simulink model "check_fence"  (Simulink 7.4)
settings: Solver=ode45  StartTime=0.0  StopTime=10.0  RelTol=1e-3
libraries: xbsIndex_r4 x293
(part 1 of 2)
settings Model: Creator=andryc  LastModifiedBy=andryc

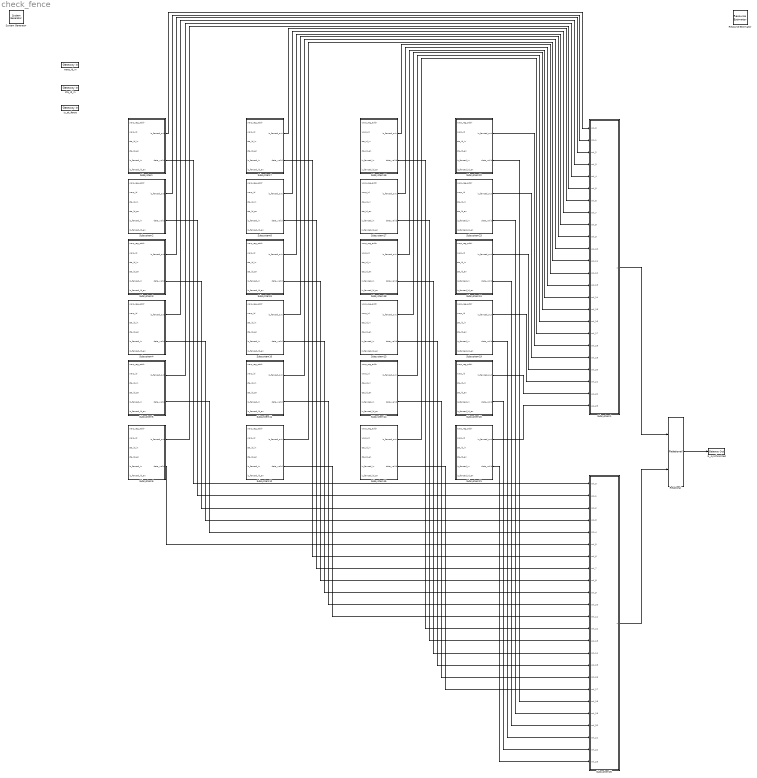
== system check_fence ==
  " System Generator" : xbsIndex_r4/ System Generator  Tag=genX  SystemSampleTime=-1  xilinxfamily=Virtex6  part=xc6vsx315t  speed=-3  package=ff1156  synthesis_tool=XST  clock_wrapper=Clock Enables  directory=./netlist  testbench=off  simulink_period=1  sysclk_period=10  dcm_input_clock_period=10  incr_netlist=off  trim_vbits=Everywhere in SubSystem  dbl_ovrd=According to Block Masks  core_generation=According to Block Masks  run_coregen=off  deprecated_control=off  eval_field=0  block_type=sysgen
  Relational : xbsIndex_r4/Relational  mode=a=b  en=off  latency=0  dbl_ovrd=off  block_type=relational
  Resource Estimator : xbsIndex_r4/Resource Estimator  Tag=resEstTag  Slices=0  FFs=0  BRAMs=0  LUTs=0  IOBs=0  EBMs=0  TBUFs=0  xl_use_estimator_area=off  est_options=Estimate  block_type=resource_estimator
      settings: AttributesFormatString=Resource\nEstimator
  Subsystem : Subsystem
  Subsystem1 : Subsystem
  Subsystem10 : Subsystem
  Subsystem11 : Subsystem
  Subsystem12 : Subsystem
  Subsystem13 : Subsystem
  Subsystem14 : Subsystem
  Subsystem15 : Subsystem
  Subsystem16 : Subsystem
  Subsystem17 : Subsystem
  Subsystem18 : Subsystem
  Subsystem19 : Subsystem
  Subsystem2 : Subsystem
  Subsystem20 : Subsystem
  Subsystem21 : Subsystem
  Subsystem22 : Subsystem
  Subsystem23 : Subsystem
  Subsystem24 : Subsystem
  Subsystem25 : Subsystem
  Subsystem3 : Subsystem
  Subsystem4 : Subsystem
  Subsystem5 : Subsystem
  Subsystem6 : Subsystem
  Subsystem7 : Subsystem
  Subsystem8 : Subsystem
  Subsystem9 : Subsystem
  cta_id_in : xbsIndex_r4/Gateway In  arith_type=Unsigned  n_bits=2  bin_pt=0  quantization=Truncate  overflow=Saturate  period=1  dbl_ovrd=off  timing_constraint=None  locs_specified=off  LOCs={}  hdl_port=on  block_type=gatewayin
      settings: infoedit="Gateway in block.  Converts inputs of type Simulink integer, double and fixed point to  Xilinx fixed point type.<br><br>Hardware notes:  In hardware these blocks become top level input ports."
  is_at_fence : xbsIndex_r4/Gateway In  arith_type=Unsigned  n_bits=2  bin_pt=0  quantization=Truncate  overflow=Saturate  period=1  dbl_ovrd=off  timing_constraint=None  locs_specified=off  LOCs={}  hdl_port=on  block_type=gatewayin
      settings: infoedit="Gateway in block.  Converts inputs of type Simulink integer, double and fixed point to  Xilinx fixed point type.<br><br>Hardware notes:  In hardware these blocks become top level input ports."
  is_synchronized : xbsIndex_r4/Gateway Out  hdl_port=on  timing_constraint=None  locs_specified=off  LOCs={}  block_type=gatewayout
      settings: infoedit="Gateway out block.  Converts Xilinx fixed point inputs into ouputs of type Simulink integer, double, or fixed point.<br><br>Hardware notes:  In hardware these blocks become top level output ports or are discarded, depending on how they are configured."
  warp_id_in : xbsIndex_r4/Gateway In  arith_type=Unsigned  n_bits=4  bin_pt=0  quantization=Truncate  overflow=Saturate  period=1  dbl_ovrd=off  timing_constraint=None  locs_specified=off  LOCs={}  hdl_port=on  block_type=gatewayin
      settings: infoedit="Gateway in block.  Converts inputs of type Simulink integer, double and fixed point to  Xilinx fixed point type.<br><br>Hardware notes:  In hardware these blocks become top level input ports."
  wires:
  Subsystem/1(is_fenced_out) -> Subsystem1/1(val_0)
  Subsystem2/1(is_fenced_out) -> Subsystem1/2(val_1)
  Subsystem3/1(is_fenced_out) -> Subsystem1/3(val_2)
  Subsystem4/1(is_fenced_out) -> Subsystem1/4(val_3)
  Subsystem5/1(is_fenced_out) -> Subsystem1/5(val_4)
  Subsystem6/1(is_fenced_out) -> Subsystem1/6(val_5)
  Subsystem7/1(is_fenced_out) -> Subsystem1/7(val_6)
  Subsystem8/1(is_fenced_out) -> Subsystem1/8(val_7)
  Subsystem9/1(is_fenced_out) -> Subsystem1/9(val_8)
  Subsystem10/1(is_fenced_out) -> Subsystem1/10(val_9)
  Subsystem11/1(is_fenced_out) -> Subsystem1/11(val_10)
  Subsystem12/1(is_fenced_out) -> Subsystem1/12(val_11)
  Subsystem16/1(is_fenced_out) -> Subsystem1/13(val_12)
  Subsystem17/1(is_fenced_out) -> Subsystem1/14(val_13)
  Subsystem18/1(is_fenced_out) -> Subsystem1/15(val_14)
  Subsystem13/1(is_fenced_out) -> Subsystem1/16(val_15)
  Subsystem14/1(is_fenced_out) -> Subsystem1/17(val_16)
  Subsystem15/1(is_fenced_out) -> Subsystem1/18(val_17)
  Subsystem22/1(is_fenced_out) -> Subsystem1/19(val_18)
  Subsystem23/1(is_fenced_out) -> Subsystem1/20(val_19)
  Subsystem24/1(is_fenced_out) -> Subsystem1/21(val_20)
  Subsystem19/1(is_fenced_out) -> Subsystem1/22(val_21)
  Subsystem20/1(is_fenced_out) -> Subsystem1/23(val_22)
  Subsystem21/1(is_fenced_out) -> Subsystem1/24(val_23)
  Subsystem/2(data_valid) -> Subsystem25/1(val_0)
  Subsystem2/2(data_valid) -> Subsystem25/2(val_1)
  Subsystem3/2(data_valid) -> Subsystem25/3(val_2)
  Subsystem4/2(data_valid) -> Subsystem25/4(val_3)
  Subsystem5/2(data_valid) -> Subsystem25/5(val_4)
  Subsystem6/2(data_valid) -> Subsystem25/6(val_5)
  Subsystem7/2(data_valid) -> Subsystem25/7(val_6)
  Subsystem8/2(data_valid) -> Subsystem25/8(val_7)
  Subsystem9/2(data_valid) -> Subsystem25/9(val_8)
  Subsystem10/2(data_valid) -> Subsystem25/10(val_9)
  Subsystem11/2(data_valid) -> Subsystem25/11(val_10)
  Subsystem12/2(data_valid) -> Subsystem25/12(val_11)
  Subsystem16/2(data_valid) -> Subsystem25/13(val_12)
  Subsystem17/2(data_valid) -> Subsystem25/14(val_13)
  Subsystem18/2(data_valid) -> Subsystem25/15(val_14)
  Subsystem13/2(data_valid) -> Subsystem25/16(val_15)
  Subsystem14/2(data_valid) -> Subsystem25/17(val_16)
  Subsystem15/2(data_valid) -> Subsystem25/18(val_17)
  Subsystem22/2(data_valid) -> Subsystem25/19(val_18)
  Subsystem23/2(data_valid) -> Subsystem25/20(val_19)
  Subsystem24/2(data_valid) -> Subsystem25/21(val_20)
  Subsystem19/2(data_valid) -> Subsystem25/22(val_21)
  Subsystem20/2(data_valid) -> Subsystem25/23(val_22)
  Subsystem21/2(data_valid) -> Subsystem25/24(val_23)
  Subsystem1/1(s) -> Relational/1
  Subsystem25/1(s) -> Relational/2
  Relational/1 -> is_synchronized/1

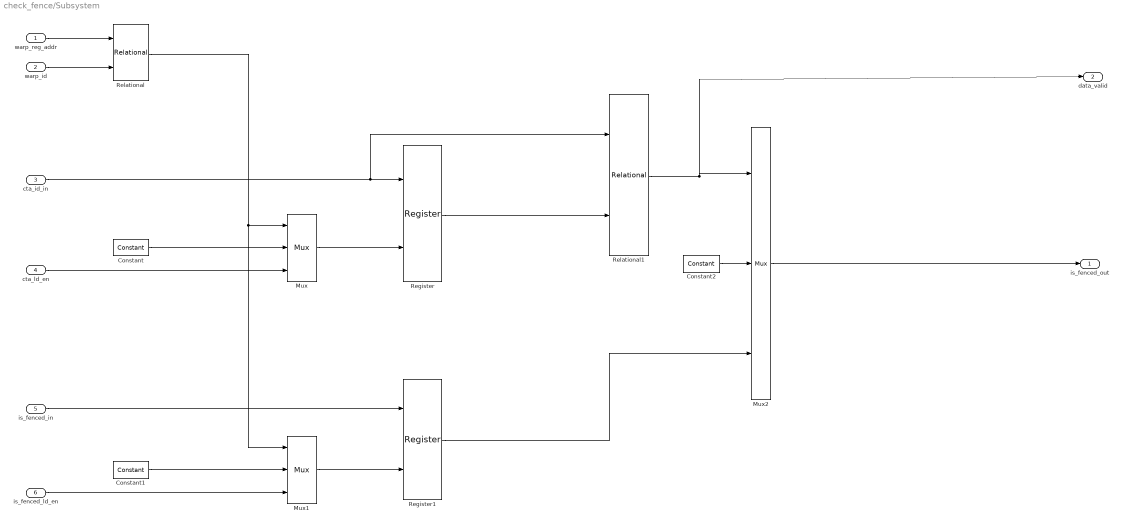
== system check_fence/Subsystem ==
  warp_reg_addr : Inport
  warp_id : Inport  Port=2
  cta_id_in : Inport  Port=3
  cta_ld_en : Inport  Port=4
  is_fenced_in : Inport  Port=5
  is_fenced_ld_en : Inport  Port=6
  Constant : xbsIndex_r4/Constant  arith_type=Boolean  const=0  n_bits=16  bin_pt=14  explicit_period=off  period=1  equ=P=C  opselect=C  inp2=PCIN>>17  opr=+  inp1=P  carry=CIN  dbl_ovrd=off  block_type=constant
  Constant1 : xbsIndex_r4/Constant  arith_type=Boolean  const=0  n_bits=16  bin_pt=14  explicit_period=off  period=1  equ=P=C  opselect=C  inp2=PCIN>>17  opr=+  inp1=P  carry=CIN  dbl_ovrd=off  block_type=constant
  Constant2 : xbsIndex_r4/Constant  arith_type=Unsigned  const=0  n_bits=1  bin_pt=0  explicit_period=off  period=1  equ=P=C  opselect=C  inp2=PCIN>>17  opr=+  inp1=P  carry=CIN  dbl_ovrd=off  block_type=constant
  Mux : xbsIndex_r4/Mux  inputs=2  en=off  latency=0  precision=Full  arith_type=Unsigned  n_bits=16  bin_pt=14  quantization=Truncate  overflow=Wrap  dbl_ovrd=off  block_type=mux
  Mux1 : xbsIndex_r4/Mux  inputs=2  en=off  latency=0  precision=Full  arith_type=Unsigned  n_bits=16  bin_pt=14  quantization=Truncate  overflow=Wrap  dbl_ovrd=off  block_type=mux
  Mux2 : xbsIndex_r4/Mux  inputs=2  en=off  latency=0  precision=Full  arith_type=Unsigned  n_bits=16  bin_pt=14  quantization=Truncate  overflow=Wrap  dbl_ovrd=off  block_type=mux
  Register : xbsIndex_r4/Register  init=0  rst=off  en=on  dbl_ovrd=off  block_type=register
  Register1 : xbsIndex_r4/Register  init=0  rst=off  en=on  dbl_ovrd=off  block_type=register
  Relational : xbsIndex_r4/Relational  mode=a=b  en=off  latency=0  dbl_ovrd=off  block_type=relational
  Relational1 : xbsIndex_r4/Relational  mode=a=b  en=off  latency=0  dbl_ovrd=off  block_type=relational
  is_fenced_out : Outport
  data_valid : Outport  Port=2
  wires:
  cta_id_in/1 -> Register/1, Relational1/1
  is_fenced_in/1 -> Register1/1
  warp_reg_addr/1 -> Relational/1
  warp_id/1 -> Relational/2
  Mux/1 -> Register/2
  cta_ld_en/1 -> Mux/3
  Constant/1 -> Mux/2
  Relational/1 -> Mux/1, Mux1/1
  Mux1/1 -> Register1/2
  is_fenced_ld_en/1 -> Mux1/3
  Constant1/1 -> Mux1/2
  Relational1/1 -> Mux2/1, data_valid/1
  Constant2/1 -> Mux2/2
  Register/1 -> Relational1/2
  Register1/1 -> Mux2/3
  Mux2/1 -> is_fenced_out/1

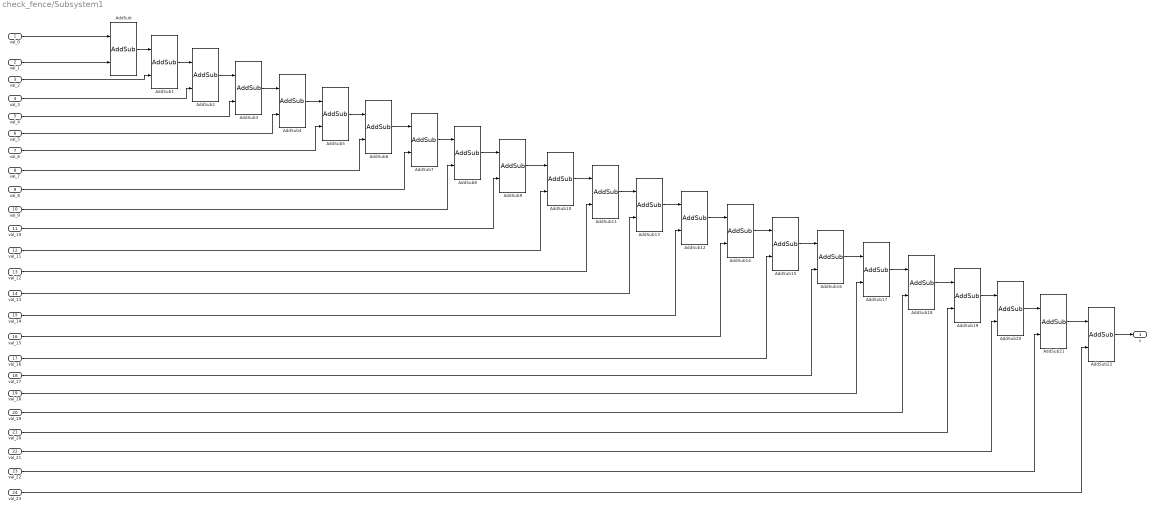
== system check_fence/Subsystem1 ==
  val_0 : Inport
  val_1 : Inport  Port=2
  val_2 : Inport  Port=3
  val_3 : Inport  Port=4
  val_4 : Inport  Port=5
  val_5 : Inport  Port=6
  val_6 : Inport  Port=7
  val_7 : Inport  Port=8
  val_8 : Inport  Port=9
  val_9 : Inport  Port=10
  val_10 : Inport  Port=11
  val_11 : Inport  Port=12
  val_12 : Inport  Port=13
  val_13 : Inport  Port=14
  val_14 : Inport  Port=15
  val_15 : Inport  Port=16
  val_16 : Inport  Port=17
  val_17 : Inport  Port=18
  val_18 : Inport  Port=19
  val_19 : Inport  Port=20
  val_20 : Inport  Port=21
  val_21 : Inport  Port=22
  val_22 : Inport  Port=23
  val_23 : Inport  Port=24
  AddSub{,1..22} (23 alike) : xbsIndex_r4/AddSub  mode=Addition  use_carryin=off  use_carryout=off  en=off  latency=0  precision=Full  arith_type=Unsigned  n_bits=16  bin_pt=14  quantization=Truncate  overflow=Wrap  dbl_ovrd=off  use_behavioral_HDL=off  hw_selection=Fabric  pipelined=off  block_type=addsub
  s : Outport
  wires:
  val_0/1 -> AddSub/1
  val_1/1 -> AddSub/2
  AddSub/1 -> AddSub1/1
  AddSub1/1 -> AddSub2/1
  AddSub2/1 -> AddSub3/1
  AddSub3/1 -> AddSub4/1
  AddSub4/1 -> AddSub5/1
  AddSub5/1 -> AddSub6/1
  AddSub6/1 -> AddSub7/1
  AddSub7/1 -> AddSub8/1
  AddSub8/1 -> AddSub9/1
  AddSub9/1 -> AddSub10/1
  AddSub10/1 -> AddSub11/1
  AddSub11/1 -> AddSub13/1
  AddSub13/1 -> AddSub12/1
  AddSub12/1 -> AddSub14/1
  AddSub14/1 -> AddSub15/1
  AddSub15/1 -> AddSub16/1
  AddSub16/1 -> AddSub17/1
  AddSub17/1 -> AddSub18/1
  AddSub18/1 -> AddSub19/1
  AddSub19/1 -> AddSub20/1
  AddSub20/1 -> AddSub21/1
  AddSub21/1 -> AddSub22/1
  AddSub22/1 -> s/1
  val_2/1 -> AddSub1/2
  val_3/1 -> AddSub2/2
  val_4/1 -> AddSub3/2
  val_5/1 -> AddSub4/2
  val_6/1 -> AddSub5/2
  val_7/1 -> AddSub6/2
  val_8/1 -> AddSub7/2
  val_9/1 -> AddSub8/2
  val_10/1 -> AddSub9/2
  val_11/1 -> AddSub10/2
  val_12/1 -> AddSub11/2
  val_13/1 -> AddSub13/2
  val_14/1 -> AddSub12/2
  val_15/1 -> AddSub14/2
  val_16/1 -> AddSub15/2
  val_17/1 -> AddSub16/2
  val_18/1 -> AddSub17/2
  val_19/1 -> AddSub18/2
  val_20/1 -> AddSub19/2
  val_21/1 -> AddSub20/2
  val_22/1 -> AddSub21/2
  val_23/1 -> AddSub22/2

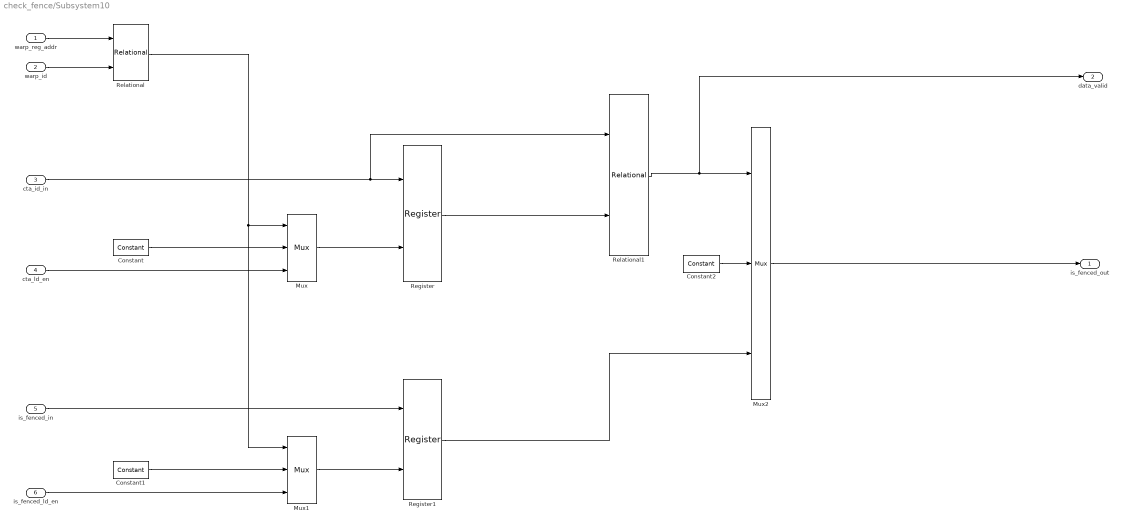
== system check_fence/Subsystem10 ==
  warp_reg_addr : Inport
  warp_id : Inport  Port=2
  cta_id_in : Inport  Port=3
  cta_ld_en : Inport  Port=4
  is_fenced_in : Inport  Port=5
  is_fenced_ld_en : Inport  Port=6
  Constant : xbsIndex_r4/Constant  arith_type=Boolean  const=0  n_bits=16  bin_pt=14  explicit_period=off  period=1  equ=P=C  opselect=C  inp2=PCIN>>17  opr=+  inp1=P  carry=CIN  dbl_ovrd=off  block_type=constant
  Constant1 : xbsIndex_r4/Constant  arith_type=Boolean  const=0  n_bits=16  bin_pt=14  explicit_period=off  period=1  equ=P=C  opselect=C  inp2=PCIN>>17  opr=+  inp1=P  carry=CIN  dbl_ovrd=off  block_type=constant
  Constant2 : xbsIndex_r4/Constant  arith_type=Unsigned  const=0  n_bits=1  bin_pt=0  explicit_period=off  period=1  equ=P=C  opselect=C  inp2=PCIN>>17  opr=+  inp1=P  carry=CIN  dbl_ovrd=off  block_type=constant
  Mux : xbsIndex_r4/Mux  inputs=2  en=off  latency=0  precision=Full  arith_type=Unsigned  n_bits=16  bin_pt=14  quantization=Truncate  overflow=Wrap  dbl_ovrd=off  block_type=mux
  Mux1 : xbsIndex_r4/Mux  inputs=2  en=off  latency=0  precision=Full  arith_type=Unsigned  n_bits=16  bin_pt=14  quantization=Truncate  overflow=Wrap  dbl_ovrd=off  block_type=mux
  Mux2 : xbsIndex_r4/Mux  inputs=2  en=off  latency=0  precision=Full  arith_type=Unsigned  n_bits=16  bin_pt=14  quantization=Truncate  overflow=Wrap  dbl_ovrd=off  block_type=mux
  Register : xbsIndex_r4/Register  init=0  rst=off  en=on  dbl_ovrd=off  block_type=register
  Register1 : xbsIndex_r4/Register  init=0  rst=off  en=on  dbl_ovrd=off  block_type=register
  Relational : xbsIndex_r4/Relational  mode=a=b  en=off  latency=0  dbl_ovrd=off  block_type=relational
  Relational1 : xbsIndex_r4/Relational  mode=a=b  en=off  latency=0  dbl_ovrd=off  block_type=relational
  is_fenced_out : Outport
  data_valid : Outport  Port=2
  wires:
  cta_id_in/1 -> Register/1, Relational1/1
  is_fenced_in/1 -> Register1/1
  warp_reg_addr/1 -> Relational/1
  warp_id/1 -> Relational/2
  Mux/1 -> Register/2
  cta_ld_en/1 -> Mux/3
  Constant/1 -> Mux/2
  Relational/1 -> Mux/1, Mux1/1
  Mux1/1 -> Register1/2
  is_fenced_ld_en/1 -> Mux1/3
  Constant1/1 -> Mux1/2
  Relational1/1 -> Mux2/1, data_valid/1
  Constant2/1 -> Mux2/2
  Register/1 -> Relational1/2
  Register1/1 -> Mux2/3
  Mux2/1 -> is_fenced_out/1

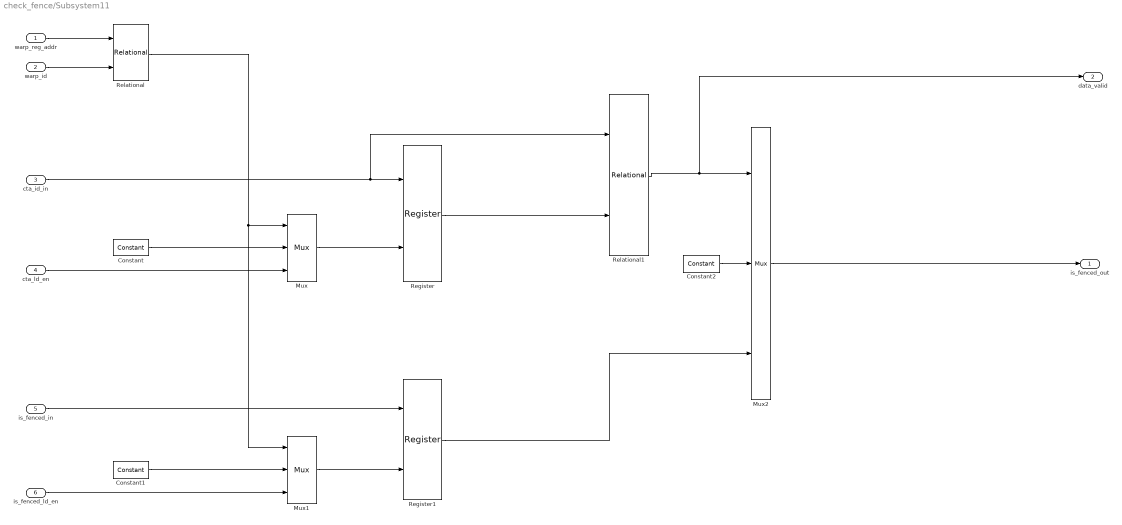
== system check_fence/Subsystem11 ==
  warp_reg_addr : Inport
  warp_id : Inport  Port=2
  cta_id_in : Inport  Port=3
  cta_ld_en : Inport  Port=4
  is_fenced_in : Inport  Port=5
  is_fenced_ld_en : Inport  Port=6
  Constant : xbsIndex_r4/Constant  arith_type=Boolean  const=0  n_bits=16  bin_pt=14  explicit_period=off  period=1  equ=P=C  opselect=C  inp2=PCIN>>17  opr=+  inp1=P  carry=CIN  dbl_ovrd=off  block_type=constant
  Constant1 : xbsIndex_r4/Constant  arith_type=Boolean  const=0  n_bits=16  bin_pt=14  explicit_period=off  period=1  equ=P=C  opselect=C  inp2=PCIN>>17  opr=+  inp1=P  carry=CIN  dbl_ovrd=off  block_type=constant
  Constant2 : xbsIndex_r4/Constant  arith_type=Unsigned  const=0  n_bits=1  bin_pt=0  explicit_period=off  period=1  equ=P=C  opselect=C  inp2=PCIN>>17  opr=+  inp1=P  carry=CIN  dbl_ovrd=off  block_type=constant
  Mux : xbsIndex_r4/Mux  inputs=2  en=off  latency=0  precision=Full  arith_type=Unsigned  n_bits=16  bin_pt=14  quantization=Truncate  overflow=Wrap  dbl_ovrd=off  block_type=mux
  Mux1 : xbsIndex_r4/Mux  inputs=2  en=off  latency=0  precision=Full  arith_type=Unsigned  n_bits=16  bin_pt=14  quantization=Truncate  overflow=Wrap  dbl_ovrd=off  block_type=mux
  Mux2 : xbsIndex_r4/Mux  inputs=2  en=off  latency=0  precision=Full  arith_type=Unsigned  n_bits=16  bin_pt=14  quantization=Truncate  overflow=Wrap  dbl_ovrd=off  block_type=mux
  Register : xbsIndex_r4/Register  init=0  rst=off  en=on  dbl_ovrd=off  block_type=register
  Register1 : xbsIndex_r4/Register  init=0  rst=off  en=on  dbl_ovrd=off  block_type=register
  Relational : xbsIndex_r4/Relational  mode=a=b  en=off  latency=0  dbl_ovrd=off  block_type=relational
  Relational1 : xbsIndex_r4/Relational  mode=a=b  en=off  latency=0  dbl_ovrd=off  block_type=relational
  is_fenced_out : Outport
  data_valid : Outport  Port=2
  wires:
  Mux2/1 -> is_fenced_out/1
  Register1/1 -> Mux2/3
  Register/1 -> Relational1/2
  Constant2/1 -> Mux2/2
  Relational1/1 -> data_valid/1, Mux2/1
  Constant1/1 -> Mux1/2
  is_fenced_ld_en/1 -> Mux1/3
  Mux1/1 -> Register1/2
  Relational/1 -> Mux1/1, Mux/1
  Constant/1 -> Mux/2
  cta_ld_en/1 -> Mux/3
  Mux/1 -> Register/2
  warp_id/1 -> Relational/2
  warp_reg_addr/1 -> Relational/1
  is_fenced_in/1 -> Register1/1
  cta_id_in/1 -> Relational1/1, Register/1

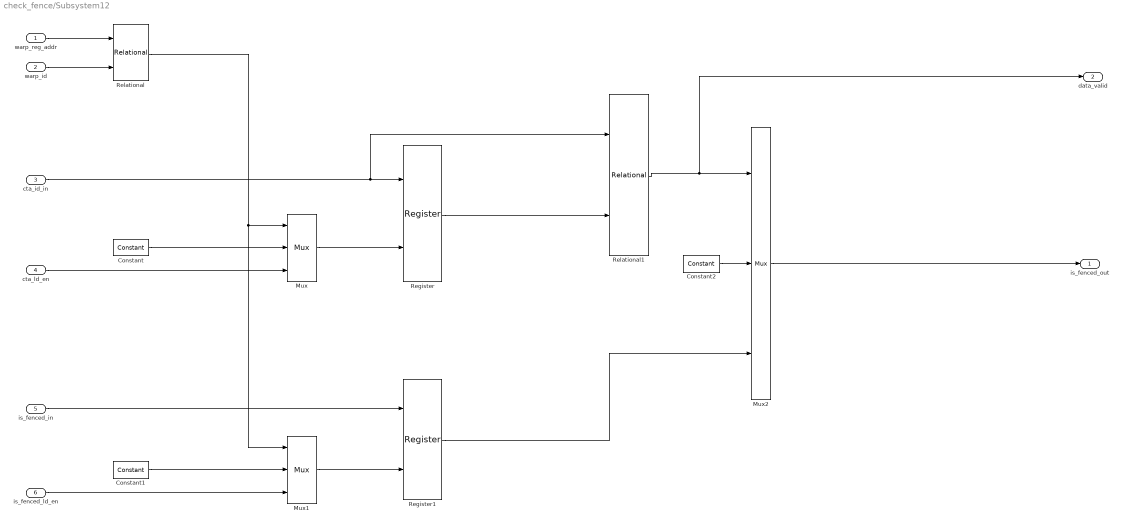
== system check_fence/Subsystem12 ==
  warp_reg_addr : Inport
  warp_id : Inport  Port=2
  cta_id_in : Inport  Port=3
  cta_ld_en : Inport  Port=4
  is_fenced_in : Inport  Port=5
  is_fenced_ld_en : Inport  Port=6
  Constant : xbsIndex_r4/Constant  arith_type=Boolean  const=0  n_bits=16  bin_pt=14  explicit_period=off  period=1  equ=P=C  opselect=C  inp2=PCIN>>17  opr=+  inp1=P  carry=CIN  dbl_ovrd=off  block_type=constant
  Constant1 : xbsIndex_r4/Constant  arith_type=Boolean  const=0  n_bits=16  bin_pt=14  explicit_period=off  period=1  equ=P=C  opselect=C  inp2=PCIN>>17  opr=+  inp1=P  carry=CIN  dbl_ovrd=off  block_type=constant
  Constant2 : xbsIndex_r4/Constant  arith_type=Unsigned  const=0  n_bits=1  bin_pt=0  explicit_period=off  period=1  equ=P=C  opselect=C  inp2=PCIN>>17  opr=+  inp1=P  carry=CIN  dbl_ovrd=off  block_type=constant
  Mux : xbsIndex_r4/Mux  inputs=2  en=off  latency=0  precision=Full  arith_type=Unsigned  n_bits=16  bin_pt=14  quantization=Truncate  overflow=Wrap  dbl_ovrd=off  block_type=mux
  Mux1 : xbsIndex_r4/Mux  inputs=2  en=off  latency=0  precision=Full  arith_type=Unsigned  n_bits=16  bin_pt=14  quantization=Truncate  overflow=Wrap  dbl_ovrd=off  block_type=mux
  Mux2 : xbsIndex_r4/Mux  inputs=2  en=off  latency=0  precision=Full  arith_type=Unsigned  n_bits=16  bin_pt=14  quantization=Truncate  overflow=Wrap  dbl_ovrd=off  block_type=mux
  Register : xbsIndex_r4/Register  init=0  rst=off  en=on  dbl_ovrd=off  block_type=register
  Register1 : xbsIndex_r4/Register  init=0  rst=off  en=on  dbl_ovrd=off  block_type=register
  Relational : xbsIndex_r4/Relational  mode=a=b  en=off  latency=0  dbl_ovrd=off  block_type=relational
  Relational1 : xbsIndex_r4/Relational  mode=a=b  en=off  latency=0  dbl_ovrd=off  block_type=relational
  is_fenced_out : Outport
  data_valid : Outport  Port=2
  wires:
  cta_id_in/1 -> Register/1, Relational1/1
  is_fenced_in/1 -> Register1/1
  warp_reg_addr/1 -> Relational/1
  warp_id/1 -> Relational/2
  Mux/1 -> Register/2
  cta_ld_en/1 -> Mux/3
  Constant/1 -> Mux/2
  Relational/1 -> Mux/1, Mux1/1
  Mux1/1 -> Register1/2
  is_fenced_ld_en/1 -> Mux1/3
  Constant1/1 -> Mux1/2
  Relational1/1 -> Mux2/1, data_valid/1
  Constant2/1 -> Mux2/2
  Register/1 -> Relational1/2
  Register1/1 -> Mux2/3
  Mux2/1 -> is_fenced_out/1

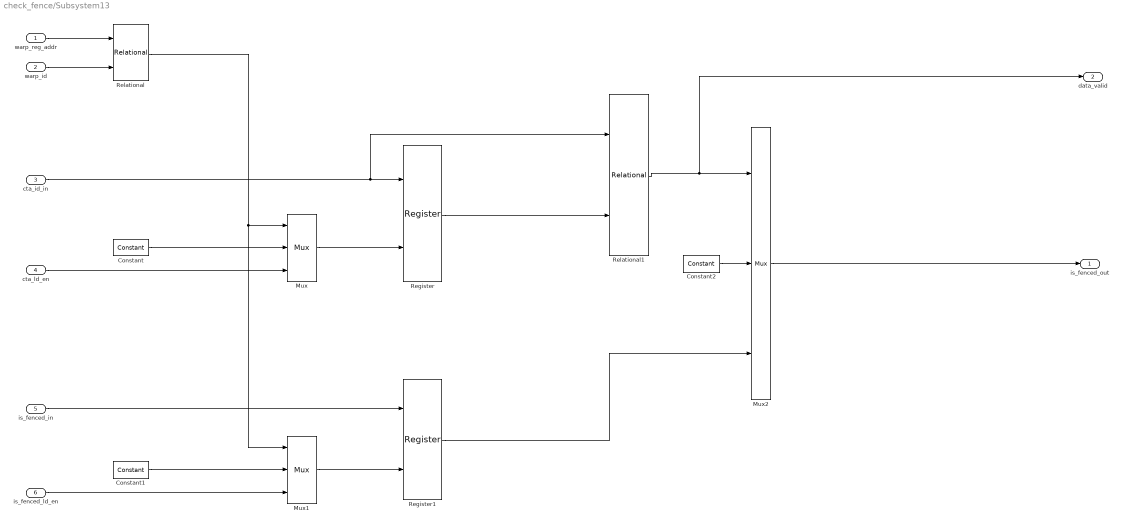
== system check_fence/Subsystem13 ==
  warp_reg_addr : Inport
  warp_id : Inport  Port=2
  cta_id_in : Inport  Port=3
  cta_ld_en : Inport  Port=4
  is_fenced_in : Inport  Port=5
  is_fenced_ld_en : Inport  Port=6
  Constant : xbsIndex_r4/Constant  arith_type=Boolean  const=0  n_bits=16  bin_pt=14  explicit_period=off  period=1  equ=P=C  opselect=C  inp2=PCIN>>17  opr=+  inp1=P  carry=CIN  dbl_ovrd=off  block_type=constant
  Constant1 : xbsIndex_r4/Constant  arith_type=Boolean  const=0  n_bits=16  bin_pt=14  explicit_period=off  period=1  equ=P=C  opselect=C  inp2=PCIN>>17  opr=+  inp1=P  carry=CIN  dbl_ovrd=off  block_type=constant
  Constant2 : xbsIndex_r4/Constant  arith_type=Unsigned  const=0  n_bits=1  bin_pt=0  explicit_period=off  period=1  equ=P=C  opselect=C  inp2=PCIN>>17  opr=+  inp1=P  carry=CIN  dbl_ovrd=off  block_type=constant
  Mux : xbsIndex_r4/Mux  inputs=2  en=off  latency=0  precision=Full  arith_type=Unsigned  n_bits=16  bin_pt=14  quantization=Truncate  overflow=Wrap  dbl_ovrd=off  block_type=mux
  Mux1 : xbsIndex_r4/Mux  inputs=2  en=off  latency=0  precision=Full  arith_type=Unsigned  n_bits=16  bin_pt=14  quantization=Truncate  overflow=Wrap  dbl_ovrd=off  block_type=mux
  Mux2 : xbsIndex_r4/Mux  inputs=2  en=off  latency=0  precision=Full  arith_type=Unsigned  n_bits=16  bin_pt=14  quantization=Truncate  overflow=Wrap  dbl_ovrd=off  block_type=mux
  Register : xbsIndex_r4/Register  init=0  rst=off  en=on  dbl_ovrd=off  block_type=register
  Register1 : xbsIndex_r4/Register  init=0  rst=off  en=on  dbl_ovrd=off  block_type=register
  Relational : xbsIndex_r4/Relational  mode=a=b  en=off  latency=0  dbl_ovrd=off  block_type=relational
  Relational1 : xbsIndex_r4/Relational  mode=a=b  en=off  latency=0  dbl_ovrd=off  block_type=relational
  is_fenced_out : Outport
  data_valid : Outport  Port=2
  wires:
  Mux2/1 -> is_fenced_out/1
  Register1/1 -> Mux2/3
  Register/1 -> Relational1/2
  Constant2/1 -> Mux2/2
  Relational1/1 -> data_valid/1, Mux2/1
  Constant1/1 -> Mux1/2
  is_fenced_ld_en/1 -> Mux1/3
  Mux1/1 -> Register1/2
  Relational/1 -> Mux1/1, Mux/1
  Constant/1 -> Mux/2
  cta_ld_en/1 -> Mux/3
  Mux/1 -> Register/2
  warp_id/1 -> Relational/2
  warp_reg_addr/1 -> Relational/1
  is_fenced_in/1 -> Register1/1
  cta_id_in/1 -> Relational1/1, Register/1

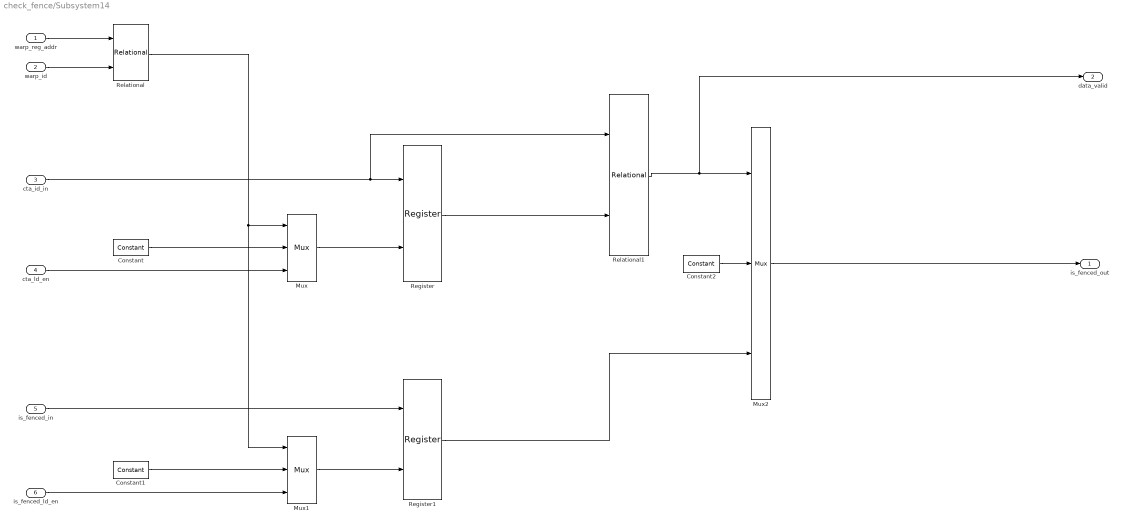
== system check_fence/Subsystem14 ==
  warp_reg_addr : Inport
  warp_id : Inport  Port=2
  cta_id_in : Inport  Port=3
  cta_ld_en : Inport  Port=4
  is_fenced_in : Inport  Port=5
  is_fenced_ld_en : Inport  Port=6
  Constant : xbsIndex_r4/Constant  arith_type=Boolean  const=0  n_bits=16  bin_pt=14  explicit_period=off  period=1  equ=P=C  opselect=C  inp2=PCIN>>17  opr=+  inp1=P  carry=CIN  dbl_ovrd=off  block_type=constant
  Constant1 : xbsIndex_r4/Constant  arith_type=Boolean  const=0  n_bits=16  bin_pt=14  explicit_period=off  period=1  equ=P=C  opselect=C  inp2=PCIN>>17  opr=+  inp1=P  carry=CIN  dbl_ovrd=off  block_type=constant
  Constant2 : xbsIndex_r4/Constant  arith_type=Unsigned  const=0  n_bits=1  bin_pt=0  explicit_period=off  period=1  equ=P=C  opselect=C  inp2=PCIN>>17  opr=+  inp1=P  carry=CIN  dbl_ovrd=off  block_type=constant
  Mux : xbsIndex_r4/Mux  inputs=2  en=off  latency=0  precision=Full  arith_type=Unsigned  n_bits=16  bin_pt=14  quantization=Truncate  overflow=Wrap  dbl_ovrd=off  block_type=mux
  Mux1 : xbsIndex_r4/Mux  inputs=2  en=off  latency=0  precision=Full  arith_type=Unsigned  n_bits=16  bin_pt=14  quantization=Truncate  overflow=Wrap  dbl_ovrd=off  block_type=mux
  Mux2 : xbsIndex_r4/Mux  inputs=2  en=off  latency=0  precision=Full  arith_type=Unsigned  n_bits=16  bin_pt=14  quantization=Truncate  overflow=Wrap  dbl_ovrd=off  block_type=mux
  Register : xbsIndex_r4/Register  init=0  rst=off  en=on  dbl_ovrd=off  block_type=register
  Register1 : xbsIndex_r4/Register  init=0  rst=off  en=on  dbl_ovrd=off  block_type=register
  Relational : xbsIndex_r4/Relational  mode=a=b  en=off  latency=0  dbl_ovrd=off  block_type=relational
  Relational1 : xbsIndex_r4/Relational  mode=a=b  en=off  latency=0  dbl_ovrd=off  block_type=relational
  is_fenced_out : Outport
  data_valid : Outport  Port=2
  wires:
  cta_id_in/1 -> Register/1, Relational1/1
  is_fenced_in/1 -> Register1/1
  warp_reg_addr/1 -> Relational/1
  warp_id/1 -> Relational/2
  Mux/1 -> Register/2
  cta_ld_en/1 -> Mux/3
  Constant/1 -> Mux/2
  Relational/1 -> Mux/1, Mux1/1
  Mux1/1 -> Register1/2
  is_fenced_ld_en/1 -> Mux1/3
  Constant1/1 -> Mux1/2
  Relational1/1 -> Mux2/1, data_valid/1
  Constant2/1 -> Mux2/2
  Register/1 -> Relational1/2
  Register1/1 -> Mux2/3
  Mux2/1 -> is_fenced_out/1

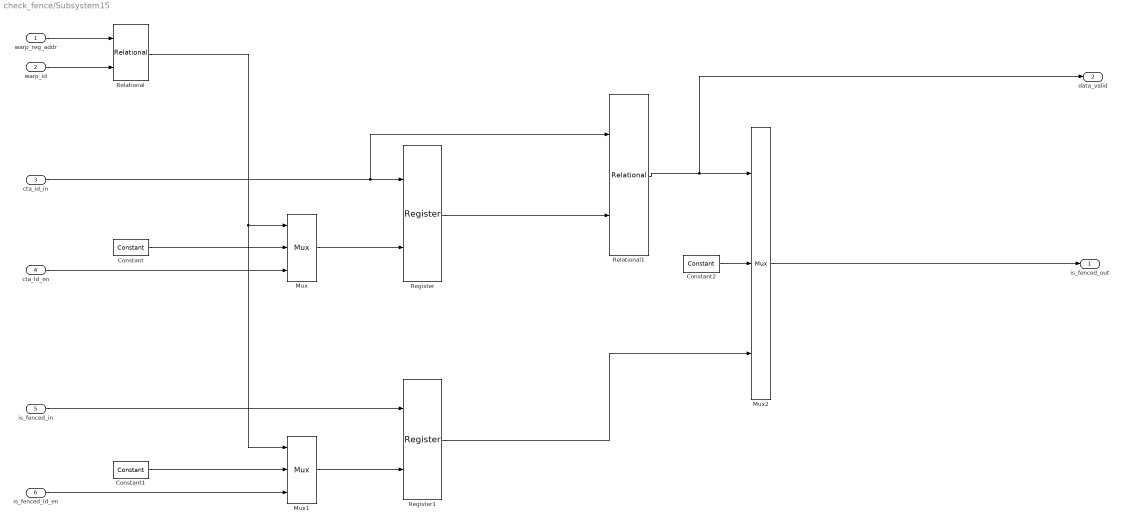
== system check_fence/Subsystem15 ==
  warp_reg_addr : Inport
  warp_id : Inport  Port=2
  cta_id_in : Inport  Port=3
  cta_ld_en : Inport  Port=4
  is_fenced_in : Inport  Port=5
  is_fenced_ld_en : Inport  Port=6
  Constant : xbsIndex_r4/Constant  arith_type=Boolean  const=0  n_bits=16  bin_pt=14  explicit_period=off  period=1  equ=P=C  opselect=C  inp2=PCIN>>17  opr=+  inp1=P  carry=CIN  dbl_ovrd=off  block_type=constant
  Constant1 : xbsIndex_r4/Constant  arith_type=Boolean  const=0  n_bits=16  bin_pt=14  explicit_period=off  period=1  equ=P=C  opselect=C  inp2=PCIN>>17  opr=+  inp1=P  carry=CIN  dbl_ovrd=off  block_type=constant
  Constant2 : xbsIndex_r4/Constant  arith_type=Unsigned  const=0  n_bits=1  bin_pt=0  explicit_period=off  period=1  equ=P=C  opselect=C  inp2=PCIN>>17  opr=+  inp1=P  carry=CIN  dbl_ovrd=off  block_type=constant
  Mux : xbsIndex_r4/Mux  inputs=2  en=off  latency=0  precision=Full  arith_type=Unsigned  n_bits=16  bin_pt=14  quantization=Truncate  overflow=Wrap  dbl_ovrd=off  block_type=mux
  Mux1 : xbsIndex_r4/Mux  inputs=2  en=off  latency=0  precision=Full  arith_type=Unsigned  n_bits=16  bin_pt=14  quantization=Truncate  overflow=Wrap  dbl_ovrd=off  block_type=mux
  Mux2 : xbsIndex_r4/Mux  inputs=2  en=off  latency=0  precision=Full  arith_type=Unsigned  n_bits=16  bin_pt=14  quantization=Truncate  overflow=Wrap  dbl_ovrd=off  block_type=mux
  Register : xbsIndex_r4/Register  init=0  rst=off  en=on  dbl_ovrd=off  block_type=register
  Register1 : xbsIndex_r4/Register  init=0  rst=off  en=on  dbl_ovrd=off  block_type=register
  Relational : xbsIndex_r4/Relational  mode=a=b  en=off  latency=0  dbl_ovrd=off  block_type=relational
  Relational1 : xbsIndex_r4/Relational  mode=a=b  en=off  latency=0  dbl_ovrd=off  block_type=relational
  is_fenced_out : Outport
  data_valid : Outport  Port=2
  wires:
  Mux2/1 -> is_fenced_out/1
  Register1/1 -> Mux2/3
  Register/1 -> Relational1/2
  Constant2/1 -> Mux2/2
  Relational1/1 -> data_valid/1, Mux2/1
  Constant1/1 -> Mux1/2
  is_fenced_ld_en/1 -> Mux1/3
  Mux1/1 -> Register1/2
  Relational/1 -> Mux1/1, Mux/1
  Constant/1 -> Mux/2
  cta_ld_en/1 -> Mux/3
  Mux/1 -> Register/2
  warp_id/1 -> Relational/2
  warp_reg_addr/1 -> Relational/1
  is_fenced_in/1 -> Register1/1
  cta_id_in/1 -> Relational1/1, Register/1

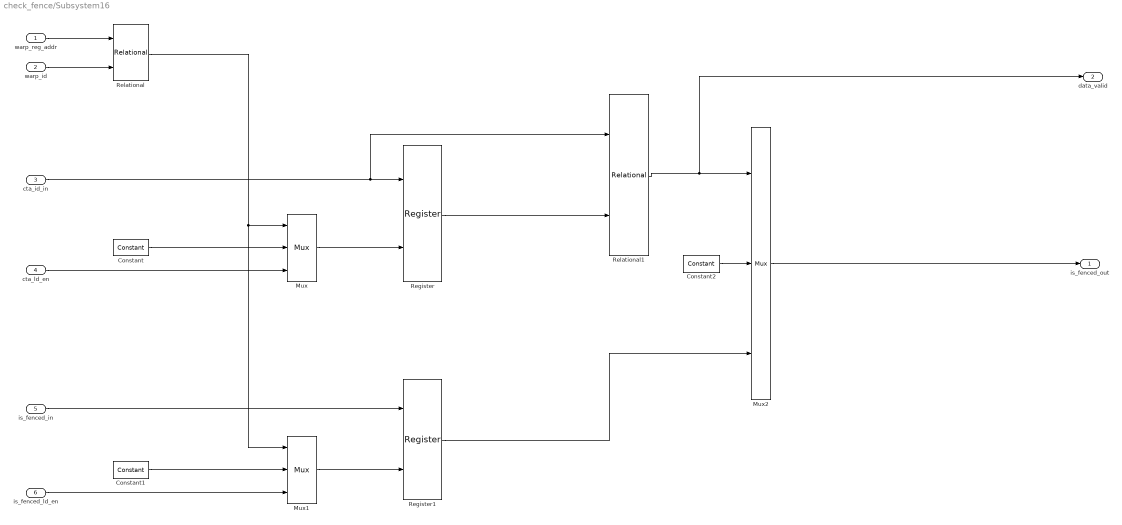
== system check_fence/Subsystem16 ==
  warp_reg_addr : Inport
  warp_id : Inport  Port=2
  cta_id_in : Inport  Port=3
  cta_ld_en : Inport  Port=4
  is_fenced_in : Inport  Port=5
  is_fenced_ld_en : Inport  Port=6
  Constant : xbsIndex_r4/Constant  arith_type=Boolean  const=0  n_bits=16  bin_pt=14  explicit_period=off  period=1  equ=P=C  opselect=C  inp2=PCIN>>17  opr=+  inp1=P  carry=CIN  dbl_ovrd=off  block_type=constant
  Constant1 : xbsIndex_r4/Constant  arith_type=Boolean  const=0  n_bits=16  bin_pt=14  explicit_period=off  period=1  equ=P=C  opselect=C  inp2=PCIN>>17  opr=+  inp1=P  carry=CIN  dbl_ovrd=off  block_type=constant
  Constant2 : xbsIndex_r4/Constant  arith_type=Unsigned  const=0  n_bits=1  bin_pt=0  explicit_period=off  period=1  equ=P=C  opselect=C  inp2=PCIN>>17  opr=+  inp1=P  carry=CIN  dbl_ovrd=off  block_type=constant
  Mux : xbsIndex_r4/Mux  inputs=2  en=off  latency=0  precision=Full  arith_type=Unsigned  n_bits=16  bin_pt=14  quantization=Truncate  overflow=Wrap  dbl_ovrd=off  block_type=mux
  Mux1 : xbsIndex_r4/Mux  inputs=2  en=off  latency=0  precision=Full  arith_type=Unsigned  n_bits=16  bin_pt=14  quantization=Truncate  overflow=Wrap  dbl_ovrd=off  block_type=mux
  Mux2 : xbsIndex_r4/Mux  inputs=2  en=off  latency=0  precision=Full  arith_type=Unsigned  n_bits=16  bin_pt=14  quantization=Truncate  overflow=Wrap  dbl_ovrd=off  block_type=mux
  Register : xbsIndex_r4/Register  init=0  rst=off  en=on  dbl_ovrd=off  block_type=register
  Register1 : xbsIndex_r4/Register  init=0  rst=off  en=on  dbl_ovrd=off  block_type=register
  Relational : xbsIndex_r4/Relational  mode=a=b  en=off  latency=0  dbl_ovrd=off  block_type=relational
  Relational1 : xbsIndex_r4/Relational  mode=a=b  en=off  latency=0  dbl_ovrd=off  block_type=relational
  is_fenced_out : Outport
  data_valid : Outport  Port=2
  wires:
  cta_id_in/1 -> Register/1, Relational1/1
  is_fenced_in/1 -> Register1/1
  warp_reg_addr/1 -> Relational/1
  warp_id/1 -> Relational/2
  Mux/1 -> Register/2
  cta_ld_en/1 -> Mux/3
  Constant/1 -> Mux/2
  Relational/1 -> Mux/1, Mux1/1
  Mux1/1 -> Register1/2
  is_fenced_ld_en/1 -> Mux1/3
  Constant1/1 -> Mux1/2
  Relational1/1 -> Mux2/1, data_valid/1
  Constant2/1 -> Mux2/2
  Register/1 -> Relational1/2
  Register1/1 -> Mux2/3
  Mux2/1 -> is_fenced_out/1

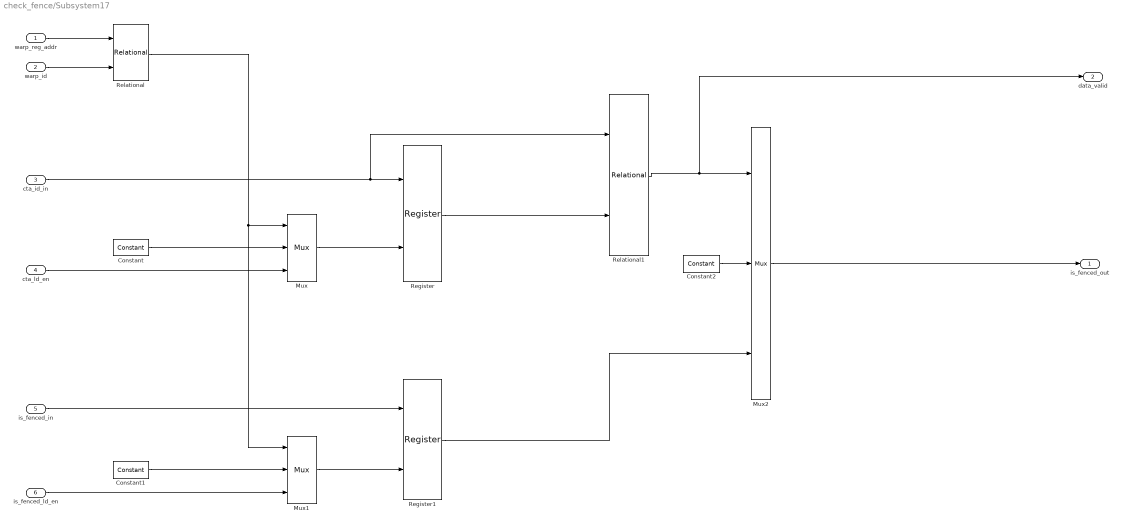
== system check_fence/Subsystem17 ==
  warp_reg_addr : Inport
  warp_id : Inport  Port=2
  cta_id_in : Inport  Port=3
  cta_ld_en : Inport  Port=4
  is_fenced_in : Inport  Port=5
  is_fenced_ld_en : Inport  Port=6
  Constant : xbsIndex_r4/Constant  arith_type=Boolean  const=0  n_bits=16  bin_pt=14  explicit_period=off  period=1  equ=P=C  opselect=C  inp2=PCIN>>17  opr=+  inp1=P  carry=CIN  dbl_ovrd=off  block_type=constant
  Constant1 : xbsIndex_r4/Constant  arith_type=Boolean  const=0  n_bits=16  bin_pt=14  explicit_period=off  period=1  equ=P=C  opselect=C  inp2=PCIN>>17  opr=+  inp1=P  carry=CIN  dbl_ovrd=off  block_type=constant
  Constant2 : xbsIndex_r4/Constant  arith_type=Unsigned  const=0  n_bits=1  bin_pt=0  explicit_period=off  period=1  equ=P=C  opselect=C  inp2=PCIN>>17  opr=+  inp1=P  carry=CIN  dbl_ovrd=off  block_type=constant
  Mux : xbsIndex_r4/Mux  inputs=2  en=off  latency=0  precision=Full  arith_type=Unsigned  n_bits=16  bin_pt=14  quantization=Truncate  overflow=Wrap  dbl_ovrd=off  block_type=mux
  Mux1 : xbsIndex_r4/Mux  inputs=2  en=off  latency=0  precision=Full  arith_type=Unsigned  n_bits=16  bin_pt=14  quantization=Truncate  overflow=Wrap  dbl_ovrd=off  block_type=mux
  Mux2 : xbsIndex_r4/Mux  inputs=2  en=off  latency=0  precision=Full  arith_type=Unsigned  n_bits=16  bin_pt=14  quantization=Truncate  overflow=Wrap  dbl_ovrd=off  block_type=mux
  Register : xbsIndex_r4/Register  init=0  rst=off  en=on  dbl_ovrd=off  block_type=register
  Register1 : xbsIndex_r4/Register  init=0  rst=off  en=on  dbl_ovrd=off  block_type=register
  Relational : xbsIndex_r4/Relational  mode=a=b  en=off  latency=0  dbl_ovrd=off  block_type=relational
  Relational1 : xbsIndex_r4/Relational  mode=a=b  en=off  latency=0  dbl_ovrd=off  block_type=relational
  is_fenced_out : Outport
  data_valid : Outport  Port=2
  wires:
  Mux2/1 -> is_fenced_out/1
  Register1/1 -> Mux2/3
  Register/1 -> Relational1/2
  Constant2/1 -> Mux2/2
  Relational1/1 -> data_valid/1, Mux2/1
  Constant1/1 -> Mux1/2
  is_fenced_ld_en/1 -> Mux1/3
  Mux1/1 -> Register1/2
  Relational/1 -> Mux1/1, Mux/1
  Constant/1 -> Mux/2
  cta_ld_en/1 -> Mux/3
  Mux/1 -> Register/2
  warp_id/1 -> Relational/2
  warp_reg_addr/1 -> Relational/1
  is_fenced_in/1 -> Register1/1
  cta_id_in/1 -> Relational1/1, Register/1

== system check_fence/Subsystem18 ==
  warp_reg_addr : Inport
  warp_id : Inport  Port=2
  cta_id_in : Inport  Port=3
  cta_ld_en : Inport  Port=4
  is_fenced_in : Inport  Port=5
  is_fenced_ld_en : Inport  Port=6
  Constant : xbsIndex_r4/Constant  arith_type=Boolean  const=0  n_bits=16  bin_pt=14  explicit_period=off  period=1  equ=P=C  opselect=C  inp2=PCIN>>17  opr=+  inp1=P  carry=CIN  dbl_ovrd=off  block_type=constant
  Constant1 : xbsIndex_r4/Constant  arith_type=Boolean  const=0  n_bits=16  bin_pt=14  explicit_period=off  period=1  equ=P=C  opselect=C  inp2=PCIN>>17  opr=+  inp1=P  carry=CIN  dbl_ovrd=off  block_type=constant
  Constant2 : xbsIndex_r4/Constant  arith_type=Unsigned  const=0  n_bits=1  bin_pt=0  explicit_period=off  period=1  equ=P=C  opselect=C  inp2=PCIN>>17  opr=+  inp1=P  carry=CIN  dbl_ovrd=off  block_type=constant
  Mux : xbsIndex_r4/Mux  inputs=2  en=off  latency=0  precision=Full  arith_type=Unsigned  n_bits=16  bin_pt=14  quantization=Truncate  overflow=Wrap  dbl_ovrd=off  block_type=mux
  Mux1 : xbsIndex_r4/Mux  inputs=2  en=off  latency=0  precision=Full  arith_type=Unsigned  n_bits=16  bin_pt=14  quantization=Truncate  overflow=Wrap  dbl_ovrd=off  block_type=mux
  Mux2 : xbsIndex_r4/Mux  inputs=2  en=off  latency=0  precision=Full  arith_type=Unsigned  n_bits=16  bin_pt=14  quantization=Truncate  overflow=Wrap  dbl_ovrd=off  block_type=mux
  Register : xbsIndex_r4/Register  init=0  rst=off  en=on  dbl_ovrd=off  block_type=register
  Register1 : xbsIndex_r4/Register  init=0  rst=off  en=on  dbl_ovrd=off  block_type=register
  Relational : xbsIndex_r4/Relational  mode=a=b  en=off  latency=0  dbl_ovrd=off  block_type=relational
  Relational1 : xbsIndex_r4/Relational  mode=a=b  en=off  latency=0  dbl_ovrd=off  block_type=relational
  is_fenced_out : Outport
  data_valid : Outport  Port=2
  wires:
  cta_id_in/1 -> Register/1, Relational1/1
  is_fenced_in/1 -> Register1/1
  warp_reg_addr/1 -> Relational/1
  warp_id/1 -> Relational/2
  Mux/1 -> Register/2
  cta_ld_en/1 -> Mux/3
  Constant/1 -> Mux/2
  Relational/1 -> Mux/1, Mux1/1
  Mux1/1 -> Register1/2
  is_fenced_ld_en/1 -> Mux1/3
  Constant1/1 -> Mux1/2
  Relational1/1 -> Mux2/1, data_valid/1
  Constant2/1 -> Mux2/2
  Register/1 -> Relational1/2
  Register1/1 -> Mux2/3
  Mux2/1 -> is_fenced_out/1

== system check_fence/Subsystem19 ==
  warp_reg_addr : Inport
  warp_id : Inport  Port=2
  cta_id_in : Inport  Port=3
  cta_ld_en : Inport  Port=4
  is_fenced_in : Inport  Port=5
  is_fenced_ld_en : Inport  Port=6
  Constant : xbsIndex_r4/Constant  arith_type=Boolean  const=0  n_bits=16  bin_pt=14  explicit_period=off  period=1  equ=P=C  opselect=C  inp2=PCIN>>17  opr=+  inp1=P  carry=CIN  dbl_ovrd=off  block_type=constant
  Constant1 : xbsIndex_r4/Constant  arith_type=Boolean  const=0  n_bits=16  bin_pt=14  explicit_period=off  period=1  equ=P=C  opselect=C  inp2=PCIN>>17  opr=+  inp1=P  carry=CIN  dbl_ovrd=off  block_type=constant
  Constant2 : xbsIndex_r4/Constant  arith_type=Unsigned  const=0  n_bits=1  bin_pt=0  explicit_period=off  period=1  equ=P=C  opselect=C  inp2=PCIN>>17  opr=+  inp1=P  carry=CIN  dbl_ovrd=off  block_type=constant
  Mux : xbsIndex_r4/Mux  inputs=2  en=off  latency=0  precision=Full  arith_type=Unsigned  n_bits=16  bin_pt=14  quantization=Truncate  overflow=Wrap  dbl_ovrd=off  block_type=mux
  Mux1 : xbsIndex_r4/Mux  inputs=2  en=off  latency=0  precision=Full  arith_type=Unsigned  n_bits=16  bin_pt=14  quantization=Truncate  overflow=Wrap  dbl_ovrd=off  block_type=mux
  Mux2 : xbsIndex_r4/Mux  inputs=2  en=off  latency=0  precision=Full  arith_type=Unsigned  n_bits=16  bin_pt=14  quantization=Truncate  overflow=Wrap  dbl_ovrd=off  block_type=mux
  Register : xbsIndex_r4/Register  init=0  rst=off  en=on  dbl_ovrd=off  block_type=register
  Register1 : xbsIndex_r4/Register  init=0  rst=off  en=on  dbl_ovrd=off  block_type=register
  Relational : xbsIndex_r4/Relational  mode=a=b  en=off  latency=0  dbl_ovrd=off  block_type=relational
  Relational1 : xbsIndex_r4/Relational  mode=a=b  en=off  latency=0  dbl_ovrd=off  block_type=relational
  is_fenced_out : Outport
  data_valid : Outport  Port=2
  wires:
  cta_id_in/1 -> Register/1, Relational1/1
  is_fenced_in/1 -> Register1/1
  warp_reg_addr/1 -> Relational/1
  warp_id/1 -> Relational/2
  Mux/1 -> Register/2
  cta_ld_en/1 -> Mux/3
  Constant/1 -> Mux/2
  Relational/1 -> Mux/1, Mux1/1
  Mux1/1 -> Register1/2
  is_fenced_ld_en/1 -> Mux1/3
  Constant1/1 -> Mux1/2
  Relational1/1 -> Mux2/1, data_valid/1
  Constant2/1 -> Mux2/2
  Register/1 -> Relational1/2
  Register1/1 -> Mux2/3
  Mux2/1 -> is_fenced_out/1

== system check_fence/Subsystem2 ==
  warp_reg_addr : Inport
  warp_id : Inport  Port=2
  cta_id_in : Inport  Port=3
  cta_ld_en : Inport  Port=4
  is_fenced_in : Inport  Port=5
  is_fenced_ld_en : Inport  Port=6
  Constant : xbsIndex_r4/Constant  arith_type=Boolean  const=0  n_bits=16  bin_pt=14  explicit_period=off  period=1  equ=P=C  opselect=C  inp2=PCIN>>17  opr=+  inp1=P  carry=CIN  dbl_ovrd=off  block_type=constant
  Constant1 : xbsIndex_r4/Constant  arith_type=Boolean  const=0  n_bits=16  bin_pt=14  explicit_period=off  period=1  equ=P=C  opselect=C  inp2=PCIN>>17  opr=+  inp1=P  carry=CIN  dbl_ovrd=off  block_type=constant
  Constant2 : xbsIndex_r4/Constant  arith_type=Unsigned  const=0  n_bits=1  bin_pt=0  explicit_period=off  period=1  equ=P=C  opselect=C  inp2=PCIN>>17  opr=+  inp1=P  carry=CIN  dbl_ovrd=off  block_type=constant
  Mux : xbsIndex_r4/Mux  inputs=2  en=off  latency=0  precision=Full  arith_type=Unsigned  n_bits=16  bin_pt=14  quantization=Truncate  overflow=Wrap  dbl_ovrd=off  block_type=mux
  Mux1 : xbsIndex_r4/Mux  inputs=2  en=off  latency=0  precision=Full  arith_type=Unsigned  n_bits=16  bin_pt=14  quantization=Truncate  overflow=Wrap  dbl_ovrd=off  block_type=mux
  Mux2 : xbsIndex_r4/Mux  inputs=2  en=off  latency=0  precision=Full  arith_type=Unsigned  n_bits=16  bin_pt=14  quantization=Truncate  overflow=Wrap  dbl_ovrd=off  block_type=mux
  Register : xbsIndex_r4/Register  init=0  rst=off  en=on  dbl_ovrd=off  block_type=register
  Register1 : xbsIndex_r4/Register  init=0  rst=off  en=on  dbl_ovrd=off  block_type=register
  Relational : xbsIndex_r4/Relational  mode=a=b  en=off  latency=0  dbl_ovrd=off  block_type=relational
  Relational1 : xbsIndex_r4/Relational  mode=a=b  en=off  latency=0  dbl_ovrd=off  block_type=relational
  is_fenced_out : Outport
  data_valid : Outport  Port=2
  wires:
  Mux2/1 -> is_fenced_out/1
  Register1/1 -> Mux2/3
  Register/1 -> Relational1/2
  Constant2/1 -> Mux2/2
  Relational1/1 -> data_valid/1, Mux2/1
  Constant1/1 -> Mux1/2
  is_fenced_ld_en/1 -> Mux1/3
  Mux1/1 -> Register1/2
  Relational/1 -> Mux1/1, Mux/1
  Constant/1 -> Mux/2
  cta_ld_en/1 -> Mux/3
  Mux/1 -> Register/2
  warp_id/1 -> Relational/2
  warp_reg_addr/1 -> Relational/1
  is_fenced_in/1 -> Register1/1
  cta_id_in/1 -> Relational1/1, Register/1

== system check_fence/Subsystem20 ==
  warp_reg_addr : Inport
  warp_id : Inport  Port=2
  cta_id_in : Inport  Port=3
  cta_ld_en : Inport  Port=4
  is_fenced_in : Inport  Port=5
  is_fenced_ld_en : Inport  Port=6
  Constant : xbsIndex_r4/Constant  arith_type=Boolean  const=0  n_bits=16  bin_pt=14  explicit_period=off  period=1  equ=P=C  opselect=C  inp2=PCIN>>17  opr=+  inp1=P  carry=CIN  dbl_ovrd=off  block_type=constant
  Constant1 : xbsIndex_r4/Constant  arith_type=Boolean  const=0  n_bits=16  bin_pt=14  explicit_period=off  period=1  equ=P=C  opselect=C  inp2=PCIN>>17  opr=+  inp1=P  carry=CIN  dbl_ovrd=off  block_type=constant
  Constant2 : xbsIndex_r4/Constant  arith_type=Unsigned  const=0  n_bits=1  bin_pt=0  explicit_period=off  period=1  equ=P=C  opselect=C  inp2=PCIN>>17  opr=+  inp1=P  carry=CIN  dbl_ovrd=off  block_type=constant
  Mux : xbsIndex_r4/Mux  inputs=2  en=off  latency=0  precision=Full  arith_type=Unsigned  n_bits=16  bin_pt=14  quantization=Truncate  overflow=Wrap  dbl_ovrd=off  block_type=mux
  Mux1 : xbsIndex_r4/Mux  inputs=2  en=off  latency=0  precision=Full  arith_type=Unsigned  n_bits=16  bin_pt=14  quantization=Truncate  overflow=Wrap  dbl_ovrd=off  block_type=mux
  Mux2 : xbsIndex_r4/Mux  inputs=2  en=off  latency=0  precision=Full  arith_type=Unsigned  n_bits=16  bin_pt=14  quantization=Truncate  overflow=Wrap  dbl_ovrd=off  block_type=mux
  Register : xbsIndex_r4/Register  init=0  rst=off  en=on  dbl_ovrd=off  block_type=register
  Register1 : xbsIndex_r4/Register  init=0  rst=off  en=on  dbl_ovrd=off  block_type=register
  Relational : xbsIndex_r4/Relational  mode=a=b  en=off  latency=0  dbl_ovrd=off  block_type=relational
  Relational1 : xbsIndex_r4/Relational  mode=a=b  en=off  latency=0  dbl_ovrd=off  block_type=relational
  is_fenced_out : Outport
  data_valid : Outport  Port=2
  wires:
  Mux2/1 -> is_fenced_out/1
  Register1/1 -> Mux2/3
  Register/1 -> Relational1/2
  Constant2/1 -> Mux2/2
  Relational1/1 -> data_valid/1, Mux2/1
  Constant1/1 -> Mux1/2
  is_fenced_ld_en/1 -> Mux1/3
  Mux1/1 -> Register1/2
  Relational/1 -> Mux1/1, Mux/1
  Constant/1 -> Mux/2
  cta_ld_en/1 -> Mux/3
  Mux/1 -> Register/2
  warp_id/1 -> Relational/2
  warp_reg_addr/1 -> Relational/1
  is_fenced_in/1 -> Register1/1
  cta_id_in/1 -> Relational1/1, Register/1

== system check_fence/Subsystem21 ==
  warp_reg_addr : Inport
  warp_id : Inport  Port=2
  cta_id_in : Inport  Port=3
  cta_ld_en : Inport  Port=4
  is_fenced_in : Inport  Port=5
  is_fenced_ld_en : Inport  Port=6
  Constant : xbsIndex_r4/Constant  arith_type=Boolean  const=0  n_bits=16  bin_pt=14  explicit_period=off  period=1  equ=P=C  opselect=C  inp2=PCIN>>17  opr=+  inp1=P  carry=CIN  dbl_ovrd=off  block_type=constant
  Constant1 : xbsIndex_r4/Constant  arith_type=Boolean  const=0  n_bits=16  bin_pt=14  explicit_period=off  period=1  equ=P=C  opselect=C  inp2=PCIN>>17  opr=+  inp1=P  carry=CIN  dbl_ovrd=off  block_type=constant
  Constant2 : xbsIndex_r4/Constant  arith_type=Unsigned  const=0  n_bits=1  bin_pt=0  explicit_period=off  period=1  equ=P=C  opselect=C  inp2=PCIN>>17  opr=+  inp1=P  carry=CIN  dbl_ovrd=off  block_type=constant
  Mux : xbsIndex_r4/Mux  inputs=2  en=off  latency=0  precision=Full  arith_type=Unsigned  n_bits=16  bin_pt=14  quantization=Truncate  overflow=Wrap  dbl_ovrd=off  block_type=mux
  Mux1 : xbsIndex_r4/Mux  inputs=2  en=off  latency=0  precision=Full  arith_type=Unsigned  n_bits=16  bin_pt=14  quantization=Truncate  overflow=Wrap  dbl_ovrd=off  block_type=mux
  Mux2 : xbsIndex_r4/Mux  inputs=2  en=off  latency=0  precision=Full  arith_type=Unsigned  n_bits=16  bin_pt=14  quantization=Truncate  overflow=Wrap  dbl_ovrd=off  block_type=mux
  Register : xbsIndex_r4/Register  init=0  rst=off  en=on  dbl_ovrd=off  block_type=register
  Register1 : xbsIndex_r4/Register  init=0  rst=off  en=on  dbl_ovrd=off  block_type=register
  Relational : xbsIndex_r4/Relational  mode=a=b  en=off  latency=0  dbl_ovrd=off  block_type=relational
  Relational1 : xbsIndex_r4/Relational  mode=a=b  en=off  latency=0  dbl_ovrd=off  block_type=relational
  is_fenced_out : Outport
  data_valid : Outport  Port=2
  wires:
  cta_id_in/1 -> Register/1, Relational1/1
  is_fenced_in/1 -> Register1/1
  warp_reg_addr/1 -> Relational/1
  warp_id/1 -> Relational/2
  Mux/1 -> Register/2
  cta_ld_en/1 -> Mux/3
  Constant/1 -> Mux/2
  Relational/1 -> Mux/1, Mux1/1
  Mux1/1 -> Register1/2
  is_fenced_ld_en/1 -> Mux1/3
  Constant1/1 -> Mux1/2
  Relational1/1 -> Mux2/1, data_valid/1
  Constant2/1 -> Mux2/2
  Register/1 -> Relational1/2
  Register1/1 -> Mux2/3
  Mux2/1 -> is_fenced_out/1

== system check_fence/Subsystem22 ==
  warp_reg_addr : Inport
  warp_id : Inport  Port=2
  cta_id_in : Inport  Port=3
  cta_ld_en : Inport  Port=4
  is_fenced_in : Inport  Port=5
  is_fenced_ld_en : Inport  Port=6
  Constant : xbsIndex_r4/Constant  arith_type=Boolean  const=0  n_bits=16  bin_pt=14  explicit_period=off  period=1  equ=P=C  opselect=C  inp2=PCIN>>17  opr=+  inp1=P  carry=CIN  dbl_ovrd=off  block_type=constant
  Constant1 : xbsIndex_r4/Constant  arith_type=Boolean  const=0  n_bits=16  bin_pt=14  explicit_period=off  period=1  equ=P=C  opselect=C  inp2=PCIN>>17  opr=+  inp1=P  carry=CIN  dbl_ovrd=off  block_type=constant
  Constant2 : xbsIndex_r4/Constant  arith_type=Unsigned  const=0  n_bits=1  bin_pt=0  explicit_period=off  period=1  equ=P=C  opselect=C  inp2=PCIN>>17  opr=+  inp1=P  carry=CIN  dbl_ovrd=off  block_type=constant
  Mux : xbsIndex_r4/Mux  inputs=2  en=off  latency=0  precision=Full  arith_type=Unsigned  n_bits=16  bin_pt=14  quantization=Truncate  overflow=Wrap  dbl_ovrd=off  block_type=mux
  Mux1 : xbsIndex_r4/Mux  inputs=2  en=off  latency=0  precision=Full  arith_type=Unsigned  n_bits=16  bin_pt=14  quantization=Truncate  overflow=Wrap  dbl_ovrd=off  block_type=mux
  Mux2 : xbsIndex_r4/Mux  inputs=2  en=off  latency=0  precision=Full  arith_type=Unsigned  n_bits=16  bin_pt=14  quantization=Truncate  overflow=Wrap  dbl_ovrd=off  block_type=mux
  Register : xbsIndex_r4/Register  init=0  rst=off  en=on  dbl_ovrd=off  block_type=register
  Register1 : xbsIndex_r4/Register  init=0  rst=off  en=on  dbl_ovrd=off  block_type=register
  Relational : xbsIndex_r4/Relational  mode=a=b  en=off  latency=0  dbl_ovrd=off  block_type=relational
  Relational1 : xbsIndex_r4/Relational  mode=a=b  en=off  latency=0  dbl_ovrd=off  block_type=relational
  is_fenced_out : Outport
  data_valid : Outport  Port=2
  wires:
  Mux2/1 -> is_fenced_out/1
  Register1/1 -> Mux2/3
  Register/1 -> Relational1/2
  Constant2/1 -> Mux2/2
  Relational1/1 -> data_valid/1, Mux2/1
  Constant1/1 -> Mux1/2
  is_fenced_ld_en/1 -> Mux1/3
  Mux1/1 -> Register1/2
  Relational/1 -> Mux1/1, Mux/1
  Constant/1 -> Mux/2
  cta_ld_en/1 -> Mux/3
  Mux/1 -> Register/2
  warp_id/1 -> Relational/2
  warp_reg_addr/1 -> Relational/1
  is_fenced_in/1 -> Register1/1
  cta_id_in/1 -> Relational1/1, Register/1

== system check_fence/Subsystem23 ==
  warp_reg_addr : Inport
  warp_id : Inport  Port=2
  cta_id_in : Inport  Port=3
  cta_ld_en : Inport  Port=4
  is_fenced_in : Inport  Port=5
  is_fenced_ld_en : Inport  Port=6
  Constant : xbsIndex_r4/Constant  arith_type=Boolean  const=0  n_bits=16  bin_pt=14  explicit_period=off  period=1  equ=P=C  opselect=C  inp2=PCIN>>17  opr=+  inp1=P  carry=CIN  dbl_ovrd=off  block_type=constant
  Constant1 : xbsIndex_r4/Constant  arith_type=Boolean  const=0  n_bits=16  bin_pt=14  explicit_period=off  period=1  equ=P=C  opselect=C  inp2=PCIN>>17  opr=+  inp1=P  carry=CIN  dbl_ovrd=off  block_type=constant
  Constant2 : xbsIndex_r4/Constant  arith_type=Unsigned  const=0  n_bits=1  bin_pt=0  explicit_period=off  period=1  equ=P=C  opselect=C  inp2=PCIN>>17  opr=+  inp1=P  carry=CIN  dbl_ovrd=off  block_type=constant
  Mux : xbsIndex_r4/Mux  inputs=2  en=off  latency=0  precision=Full  arith_type=Unsigned  n_bits=16  bin_pt=14  quantization=Truncate  overflow=Wrap  dbl_ovrd=off  block_type=mux
  Mux1 : xbsIndex_r4/Mux  inputs=2  en=off  latency=0  precision=Full  arith_type=Unsigned  n_bits=16  bin_pt=14  quantization=Truncate  overflow=Wrap  dbl_ovrd=off  block_type=mux
  Mux2 : xbsIndex_r4/Mux  inputs=2  en=off  latency=0  precision=Full  arith_type=Unsigned  n_bits=16  bin_pt=14  quantization=Truncate  overflow=Wrap  dbl_ovrd=off  block_type=mux
  Register : xbsIndex_r4/Register  init=0  rst=off  en=on  dbl_ovrd=off  block_type=register
  Register1 : xbsIndex_r4/Register  init=0  rst=off  en=on  dbl_ovrd=off  block_type=register
  Relational : xbsIndex_r4/Relational  mode=a=b  en=off  latency=0  dbl_ovrd=off  block_type=relational
  Relational1 : xbsIndex_r4/Relational  mode=a=b  en=off  latency=0  dbl_ovrd=off  block_type=relational
  is_fenced_out : Outport
  data_valid : Outport  Port=2
  wires:
  cta_id_in/1 -> Register/1, Relational1/1
  is_fenced_in/1 -> Register1/1
  warp_reg_addr/1 -> Relational/1
  warp_id/1 -> Relational/2
  Mux/1 -> Register/2
  cta_ld_en/1 -> Mux/3
  Constant/1 -> Mux/2
  Relational/1 -> Mux/1, Mux1/1
  Mux1/1 -> Register1/2
  is_fenced_ld_en/1 -> Mux1/3
  Constant1/1 -> Mux1/2
  Relational1/1 -> Mux2/1, data_valid/1
  Constant2/1 -> Mux2/2
  Register/1 -> Relational1/2
  Register1/1 -> Mux2/3
  Mux2/1 -> is_fenced_out/1

== system check_fence/Subsystem24 ==
  warp_reg_addr : Inport
  warp_id : Inport  Port=2
  cta_id_in : Inport  Port=3
  cta_ld_en : Inport  Port=4
  is_fenced_in : Inport  Port=5
  is_fenced_ld_en : Inport  Port=6
  Constant : xbsIndex_r4/Constant  arith_type=Boolean  const=0  n_bits=16  bin_pt=14  explicit_period=off  period=1  equ=P=C  opselect=C  inp2=PCIN>>17  opr=+  inp1=P  carry=CIN  dbl_ovrd=off  block_type=constant
  Constant1 : xbsIndex_r4/Constant  arith_type=Boolean  const=0  n_bits=16  bin_pt=14  explicit_period=off  period=1  equ=P=C  opselect=C  inp2=PCIN>>17  opr=+  inp1=P  carry=CIN  dbl_ovrd=off  block_type=constant
  Constant2 : xbsIndex_r4/Constant  arith_type=Unsigned  const=0  n_bits=1  bin_pt=0  explicit_period=off  period=1  equ=P=C  opselect=C  inp2=PCIN>>17  opr=+  inp1=P  carry=CIN  dbl_ovrd=off  block_type=constant
  Mux : xbsIndex_r4/Mux  inputs=2  en=off  latency=0  precision=Full  arith_type=Unsigned  n_bits=16  bin_pt=14  quantization=Truncate  overflow=Wrap  dbl_ovrd=off  block_type=mux
  Mux1 : xbsIndex_r4/Mux  inputs=2  en=off  latency=0  precision=Full  arith_type=Unsigned  n_bits=16  bin_pt=14  quantization=Truncate  overflow=Wrap  dbl_ovrd=off  block_type=mux
  Mux2 : xbsIndex_r4/Mux  inputs=2  en=off  latency=0  precision=Full  arith_type=Unsigned  n_bits=16  bin_pt=14  quantization=Truncate  overflow=Wrap  dbl_ovrd=off  block_type=mux
  Register : xbsIndex_r4/Register  init=0  rst=off  en=on  dbl_ovrd=off  block_type=register
  Register1 : xbsIndex_r4/Register  init=0  rst=off  en=on  dbl_ovrd=off  block_type=register
  Relational : xbsIndex_r4/Relational  mode=a=b  en=off  latency=0  dbl_ovrd=off  block_type=relational
  Relational1 : xbsIndex_r4/Relational  mode=a=b  en=off  latency=0  dbl_ovrd=off  block_type=relational
  is_fenced_out : Outport
  data_valid : Outport  Port=2
  wires:
  Mux2/1 -> is_fenced_out/1
  Register1/1 -> Mux2/3
  Register/1 -> Relational1/2
  Constant2/1 -> Mux2/2
  Relational1/1 -> data_valid/1, Mux2/1
  Constant1/1 -> Mux1/2
  is_fenced_ld_en/1 -> Mux1/3
  Mux1/1 -> Register1/2
  Relational/1 -> Mux1/1, Mux/1
  Constant/1 -> Mux/2
  cta_ld_en/1 -> Mux/3
  Mux/1 -> Register/2
  warp_id/1 -> Relational/2
  warp_reg_addr/1 -> Relational/1
  is_fenced_in/1 -> Register1/1
  cta_id_in/1 -> Relational1/1, Register/1
